simulink model "noise11"  (Simulink 8.1)
settings: Solver=FixedStepDiscrete  StartTime=0.0  StopTime=4.99  FixedStep=1/22050  RelTol=1e-3
InitFcn:
  | global y1;
model workspace: external: MAT-File speech_dft.mat (data not in the file)
values from neighbouring files (symbols this model uses):
  fs = 16000    [test_nn.m]    (also in training_code_new.m)
undefined symbols (not defined in the file or in its folder): magnitude, Newton, Raphson
libraries: dspxfrm3 x2, dspsigops x1
settings Model: Creator=The MathWorks Inc.  LastModifiedBy=user  ExtModeTrigMode=oneshot  ExtModeArmWhenConnect=off  ExtModeAutoUpdateStatusClock=off
settings DataIOCC: LimitDataPoints=off  SaveOutput=off  SaveTime=off  SignalLoggingName=sigsOut
settings OptimizationCC: InlineParams=on  InlineInvariantSignals=on  InitFltsAndDblsToZero=on
settings DebuggingCC: SaveWithParameterizedLinksMsg=none  CheckExecutionContextPreStartOutputMsg=on  CheckExecutionContextRuntimeOutputMsg=on  SignalResolutionControl=TryResolveAllWithWarning  SolverPrmCheckMsg=none  MultiTaskDSMMsg=warning  MultiTaskCondExecSysMsg=none  StrictBusMsg=None
settings HardwareCC: ProdHWDeviceType=Specified  TargetUnknown=on
settings RTWCC: IncludeERTFirstTime=on
settings GRTTargetCC: TargetFcnLib=ansi_tfl_tmw.mat

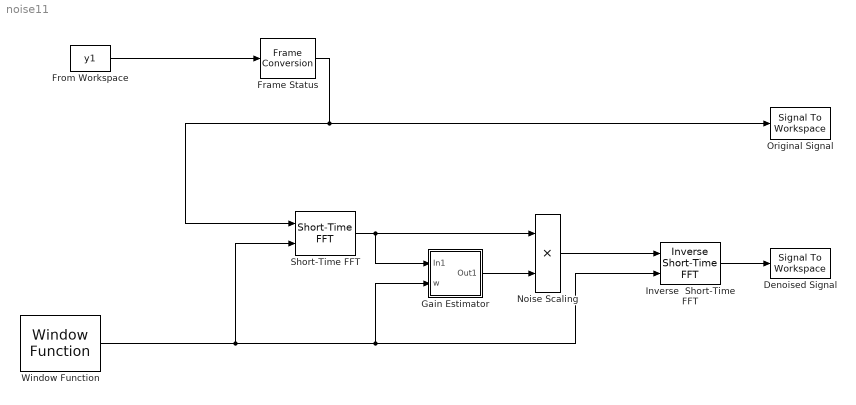
== system noise11 ==
  Denoised Signal : SignalToWorkspace  VariableName=outSig
  Frame Status : FrameConversion
  From Workspace : FromWorkspace  VariableName=y1  SampleTime=1/fs  Interpolate=off  OutputAfterFinalValue=Setting to zero
  Gain Estimator : Subsystem  mask(Estimate Gain for Noise Suppression){noiseStd=0.05, decimat=16, alpha=15}
      mask prompts: noiseStd "Noise Standard Deviation:"; decimat "Decimation:"; alpha "Weighting (alpha):"
      mask Display: disp(sprintf('Gain\n Estimator'))
  Inverse  Short-Time FFT : dspxfrm3/Inverse  Short-Time FFT  W=512  OvLap=512-16  OutFrameSize=512  InConjSymm=on  DoAssert=off  Tol=1e-4
  Noise Scaling : Product  InputSameDT=on  OutDataTypeStr=Inherit: Same as first input
  Original Signal : SignalToWorkspace  VariableName=originalSig
  Short-Time FFT : dspxfrm3/Short-Time FFT  W=512  OvLap=512-16  M=1024  TreatMby1Signals=One channel
  Window Function : dspsigops/Window Function  winmode=Generate window  wintype=Hamming  sampmode=Discrete  samptime=inf  N=512  Rs=50  beta=10  winsamp=Symmetric  UserWindow=hamming  OptParams=off  UserParams={'symmetric'}  RowConvenienceOn=on  dataType=double  isSigned=on  wordLen=16  udDataType=sfix(16)  fracBitsMode=Best precision  numFracBits=15  roundingMode=Floor  overflowMode=off  numSidelobes=4  sidelobeLevel=-30
  wires:
  Frame Status/1 -> Short-Time FFT/1, Original Signal/1
  Window Function/1 -> Gain Estimator/2(w), Inverse  Short-Time FFT/2, Short-Time FFT/2
  Inverse  Short-Time FFT/1 -> Denoised Signal/1
  Noise Scaling/1 -> Inverse  Short-Time FFT/1
  Short-Time FFT/1 -> Noise Scaling/1, Gain Estimator/1(In1)
  Gain Estimator/1(Out1) -> Noise Scaling/2
  From Workspace/1 -> Frame Status/1

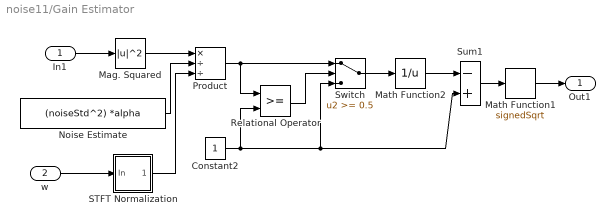
== system noise11/Gain Estimator ==
  In1 : Inport
  w : Inport  Port=2
  Constant2 : Constant
  Mag. Squared : Math  Operator=magnitude^2  SaturateOnIntegerOverflow=on
  Math Function1 : Sqrt  Operator=signedSqrt  AlgorithmType=Newton-Raphson  SaturateOnIntegerOverflow=on
  Math Function2 : Math  Operator=reciprocal  SaturateOnIntegerOverflow=on
  Noise Estimate : Constant  Value=(noiseStd^2) *alpha
  Product : Product  Inputs=*//  SaturateOnIntegerOverflow=on  InputSameDT=on  OutDataTypeStr=Inherit: Same as first input
  Relational Operator : RelationalOperator  InputSameDT=on
  STFT Normalization : Subsystem
  Sum1 : Sum  Inputs=-+  SaturateOnIntegerOverflow=on  InputSameDT=on  OutDataTypeStr=Inherit: Same as first input
  Switch : Switch  Threshold=0.5  SaturateOnIntegerOverflow=on  InputSameDT=on
  Out1 : Outport
  wires:
  Mag. Squared/1 -> Product/1
  In1/1 -> Mag. Squared/1
  Noise Estimate/1 -> Product/2
  Constant2/1 -> Relational Operator/2, Switch/3, Sum1/2
  Switch/1 -> Math Function2/1
  Relational Operator/1 -> Switch/2
  Product/1 -> Relational Operator/1, Switch/1
  Math Function2/1 -> Sum1/1
  Math Function1/1 -> Out1/1
  Sum1/1 -> Math Function1/1
  w/1 -> STFT Normalization/1(In)
  STFT Normalization/1(Out) -> Product/3

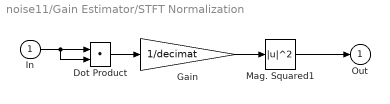
== system noise11/Gain Estimator/STFT Normalization ==
  In : Inport
  Dot Product : DotProduct  OutDataTypeStr=Inherit: Inherit via internal rule
  Gain : Gain  Gain=1/decimat  SaturateOnIntegerOverflow=on  OutDataTypeStr=Inherit: Same as input  ParamDataTypeStr=Inherit: Same as input
  Mag. Squared1 : Math  Operator=magnitude^2  SaturateOnIntegerOverflow=on
  Out : Outport
  wires:
  Dot Product/1 -> Gain/1
  In/1 -> Dot Product/1, Dot Product/2
  Gain/1 -> Mag. Squared1/1
  Mag. Squared1/1 -> Out/1
